simulink model "System_model"  (R2025a)
settings: Solver=VariableStepAuto  StartTime=0.0  StopTime=30.0  RelTol=1e-3
settings Model: Creator=chris  LastModifiedBy=chris

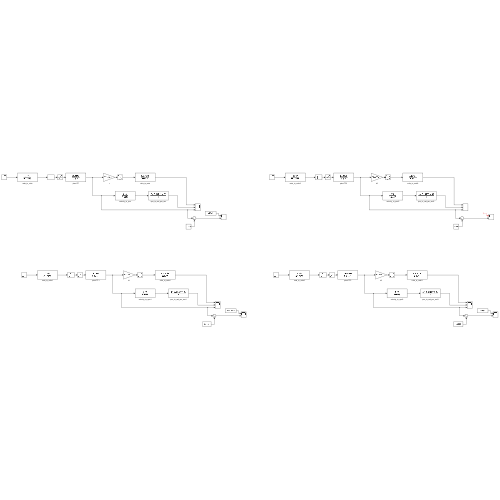
[thumbnail: Simulink's stored preview of the top-level diagram]
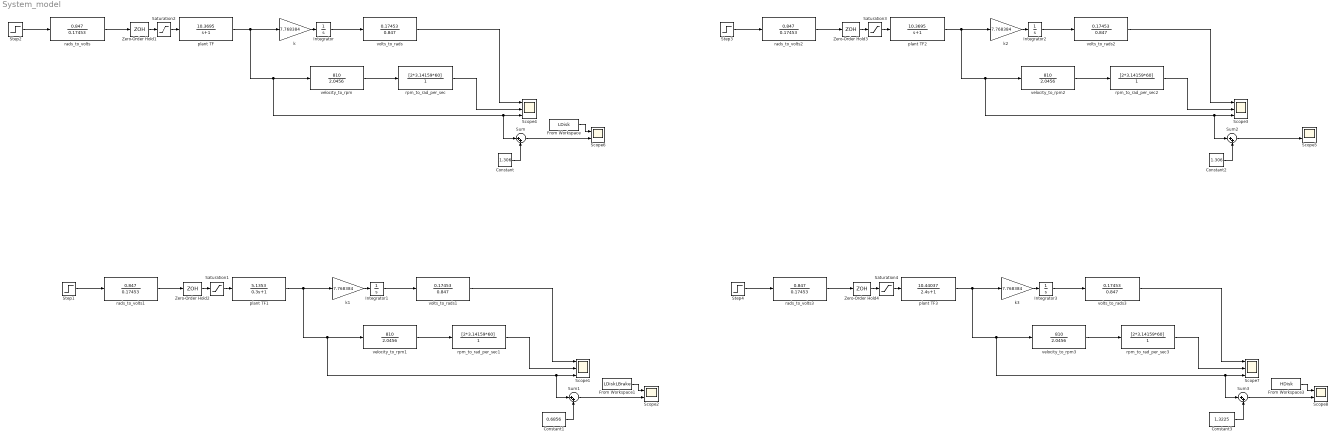
== system System_model ==
  Constant : Constant  Value=1.306
  Constant1 : Constant  Value=0.6856
  Constant2 : Constant  Value=1.306
  Constant3 : Constant  Value=1.3225
  From Workspace : FromWorkspace  VariableName=LDisk
  From Workspace1 : FromWorkspace  VariableName=LDiskLBrake
  From Workspace3 : FromWorkspace  VariableName=HDisk
  Integrator{,1..3} (4 alike) : Integrator  WrapState=on  WrappedStateUpperValue=5  WrappedStateLowerValue=-5
  Saturation{1..4} (4 alike) : Saturate  UpperLimit=10  LowerLimit=-10
  Scope{1,3..4,7} (4 alike) : Scope  NumInputPorts=3
      Scope1 settings: ActiveDisplayYMinimum=-0.64789538725322571  ActiveDisplayYMaximum=5.8310584852790326
      Scope3 settings: ActiveDisplayYMinimum=-0.64789538725322571  ActiveDisplayYMaximum=5.8310584852790326  DataLoggingVariableName=ScopeData2
      Scope4 settings: ActiveDisplayYMinimum=-0.64789538725322571  ActiveDisplayYMaximum=5.8310584852790326  DataLoggingVariableName=ScopeData4
      Scope7 settings: ActiveDisplayYMinimum=-0.64789538725322571  ActiveDisplayYMaximum=5.8310584852790326  DataLoggingVariableName=ScopeData5
  Scope{2,5..6,8} (4 alike) : Scope  NumInputPorts=2
      Scope2 settings: ActiveDisplayYMinimum=-0.38001899076662404  ActiveDisplayYMaximum=10.67968012002196
      Scope5 settings: ActiveDisplayYMinimum=-0.38001899076662404  ActiveDisplayYMaximum=10.67968012002196  DataLoggingVariableName=ScopeData3
      Scope6 settings: ActiveDisplayYMinimum=-0.38001899076662404  ActiveDisplayYMaximum=10.67968012002196  DataLoggingVariableName=ScopeData6
      Scope8 settings: ActiveDisplayYMinimum=-0.66222291272755651  ActiveDisplayYMaximum=11.531095356916857  DataLoggingVariableName=ScopeData7
  Step1 : Step  Time=13.6  After=0.103  SampleTime=0
  Step2 : Step  Time=17.2  After=0.103  SampleTime=0
  Step3 : Step  Time=17.2  After=0.103  SampleTime=0
  Step4 : Step  Time=19.6  After=0.103  SampleTime=0
  Sum{,1..3} (4 alike) : Sum  Inputs=|++
  Zero-Order Hold{1..4} (4 alike) : ZeroOrderHold  SampleTime=-1
  k{,1..3} (4 alike) : Gain  Gain=7.768384
  plant TF : TransferFcn  Numerator=[10.3695]  Denominator=[1 1]
  plant TF1 : TransferFcn  Numerator=[5.1353]  Denominator=[0.3 1]
  plant TF2 : TransferFcn  Numerator=[10.3695]  Denominator=[1 1]
  plant TF3 : TransferFcn  Numerator=[10.44037]  Denominator=[2.4 1]
  rads_to_volts{,1..3} (4 alike) : TransferFcn  Numerator=[0.847]  Denominator=[0 0.17453]
  rpm_to_rad_per_sec{,1..3} (4 alike) : TransferFcn  Numerator=[2*3.14159*60]  Denominator=[ 1]
  velocity_to_rpm{,1..3} (4 alike) : TransferFcn  Numerator=[810]  Denominator=[0 2.0456]
  volts_to_rads{,1..3} (4 alike) : TransferFcn  Numerator=[0.17453]  Denominator=[0 0.847]
  wires:
  volts_to_rads/1 -> Scope4/1
  Step2/1 -> rads_to_volts/1
  Zero-Order Hold1/1 -> Saturation2/1
  Saturation2/1 -> plant TF/1
  k/1 -> Integrator/1
  rads_to_volts/1 -> Zero-Order Hold1/1
  velocity_to_rpm/1 -> rpm_to_rad_per_sec/1
  rpm_to_rad_per_sec/1 -> Scope4/2
  Integrator/1 -> volts_to_rads/1
  Constant/1 -> Sum/2
  Sum/1 -> Scope6/2
  plant TF/1 -> k/1, Sum/1, Scope4/3, velocity_to_rpm/1
  From Workspace/1 -> Scope6/1
  volts_to_rads1/1 -> Scope1/1
  rpm_to_rad_per_sec1/1 -> Scope1/2
  From Workspace1/1 -> Scope2/1
  velocity_to_rpm1/1 -> rpm_to_rad_per_sec1/1
  Zero-Order Hold2/1 -> Saturation1/1
  Sum1/1 -> Scope2/2
  Integrator1/1 -> volts_to_rads1/1
  plant TF1/1 -> k1/1, Sum1/1, Scope1/3, velocity_to_rpm1/1
  Saturation1/1 -> plant TF1/1
  k1/1 -> Integrator1/1
  Constant1/1 -> Sum1/2
  Step1/1 -> rads_to_volts1/1
  rads_to_volts1/1 -> Zero-Order Hold2/1
  volts_to_rads2/1 -> Scope3/1
  rpm_to_rad_per_sec2/1 -> Scope3/2
  ? -> Scope5/1
  velocity_to_rpm2/1 -> rpm_to_rad_per_sec2/1
  Zero-Order Hold3/1 -> Saturation3/1
  Sum2/1 -> Scope5/2
  Integrator2/1 -> volts_to_rads2/1
  plant TF2/1 -> k2/1, Sum2/1, Scope3/3, velocity_to_rpm2/1
  Saturation3/1 -> plant TF2/1
  k2/1 -> Integrator2/1
  Constant2/1 -> Sum2/2
  Step3/1 -> rads_to_volts2/1
  rads_to_volts2/1 -> Zero-Order Hold3/1
  volts_to_rads3/1 -> Scope7/1
  rpm_to_rad_per_sec3/1 -> Scope7/2
  From Workspace3/1 -> Scope8/1
  velocity_to_rpm3/1 -> rpm_to_rad_per_sec3/1
  Zero-Order Hold4/1 -> Saturation4/1
  Sum3/1 -> Scope8/2
  Integrator3/1 -> volts_to_rads3/1
  plant TF3/1 -> k3/1, Sum3/1, Scope7/3, velocity_to_rpm3/1
  Saturation4/1 -> plant TF3/1
  k3/1 -> Integrator3/1
  Constant3/1 -> Sum3/2
  Step4/1 -> rads_to_volts3/1
  rads_to_volts3/1 -> Zero-Order Hold4/1
